simulink model "Control_Unit"  (R2023b)
settings: Solver=ode1  StartTime=0.0  StopTime=100  FixedStep=0.02  RelTol=1e-3  AbsTol=1e-3  EnableMultiTasking=on
model workspace: external: MATLAB File model_workspace.m (data not in the file)
values from neighbouring files (symbols this model uses):
  time_step = 0.02    [model_workspace.m]
libraries: slpidlib x3
settings Model: Creator=The MathWorks, Inc.  LastModifiedBy=danie
settings ConfigSet: Description=VeriStand Targets (Windows & NI Linux Real-Time 64-bit)
settings SolverCC: AutoScaleAbsTol=off  MaxConsecutiveMinStep=2  AlgebraicLoopSolver=TrustRegion  AutoInsertRateTranBlk=on  InsertRTBMode=Always  MaxZcPerStep=1
settings DataIOCC: SaveOutput=off  SaveTime=off  ReturnWorkspaceOutputs=off
settings OptimizationCC: DefaultParameterBehavior=Inlined  EnhancedBackFolding=on  PassReuseOutputArgsAs=Individual arguments  ZeroExternalMemoryAtStartup=off  ZeroInternalMemoryAtStartup=off  OptimizeBlockOrder=speed  DifferentSizesBufferReuse=on  OptimizationCustomize=off  EfficientTunableParamExpr=on
settings DebuggingCC: ParameterTunabilityLossMsg=error  UnconnectedInputMsg=warning  UnconnectedOutputMsg=warning  UnconnectedLineMsg=warning  SymbolicDimsDataTypeCodeGenerationDiagnostic=none
settings HardwareCC: ProdBitPerLong=64  ProdHWDeviceType=Intel->x86-64 (Linux 64)
settings ModelReferenceCC: EnableRefExpFcnMdlSchedulingChecks=on
settings SFSimCC: MATLABDynamicMemAlloc=off  CustomCodeUndefinedFunction=UseInterfaceOnly
settings RTWCC: Description=Embedded Coder  SystemTargetFile=ert.tlc  GenCodeOnly=on  PackageGeneratedCodeAndArtifacts=on  TemplateMakefile=ert_default_tmf  BuildConfiguration=Faster Runs  DLArmComputeVersion=19.05
settings CodeAppCC: ForceParamTrailComments=on  IgnoreCustomStorageClasses=off  OperatorAnnotations=on  SimulinkDataObjDesc=on  SFDataObjDesc=on  InsertBlockDesc=on
settings ERTTargetCC: TargetLangStandard=C99 (ISO)  GenerateSampleERTMain=on  InlinedParameterPlacement=NonHierarchical  ERTCustomFileTemplate=example_file_process.tlc
settings SimscapeCC: SimscapeLogType=all  SimscapeLogSimulationStatistics=on  SimscapeLogName=simlog_ssc_fuel_cell  SimscapeLogDataHistory=20000

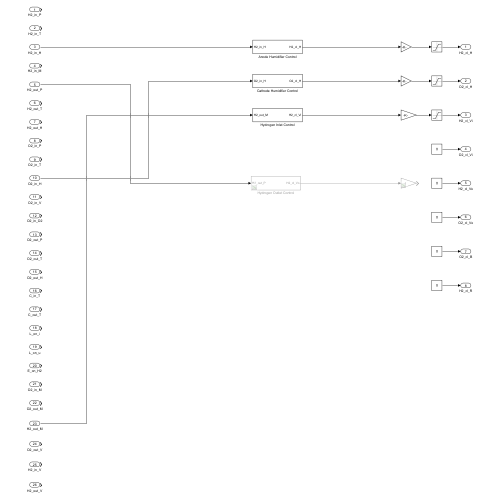
[thumbnail: Simulink's stored preview of the top-level diagram]
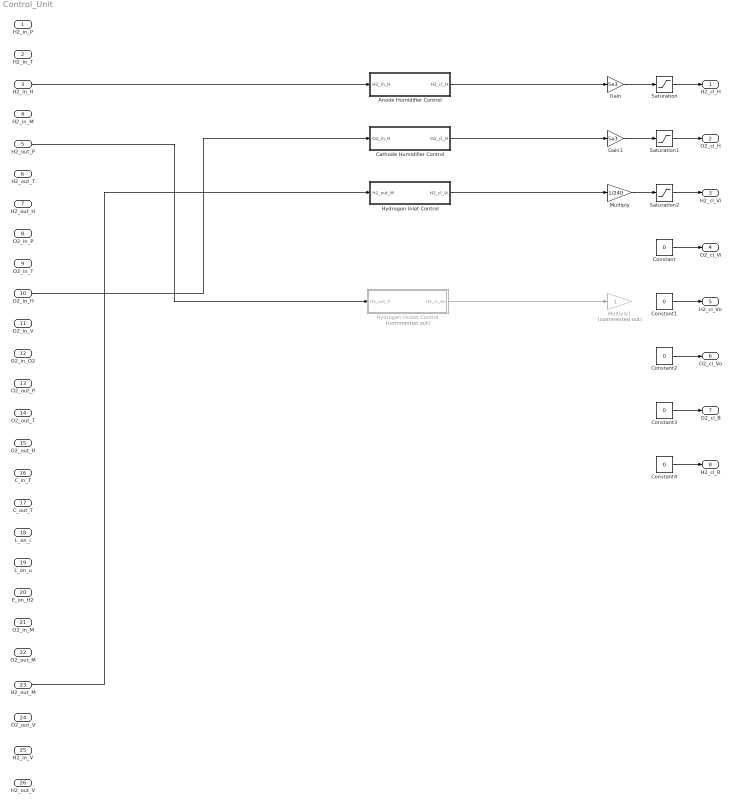
== system Control_Unit ==
  H2_in_P : Inport  OutDataTypeStr=double  PortDimensions=[1 1]  SampleTime=[time_step,0]
  H2_in_T : Inport  Port=2  OutDataTypeStr=double  PortDimensions=[1 1]  SampleTime=[time_step,0]
  H2_in_H : Inport  Port=3  OutDataTypeStr=double  PortDimensions=[1 1]  SampleTime=[time_step,0]
  H2_in_M : Inport  Port=4  OutDataTypeStr=double  PortDimensions=[1 1]  SampleTime=[time_step,0]
  H2_out_P : Inport  Port=5  OutDataTypeStr=double  PortDimensions=[1 1]  SampleTime=[time_step,0]
  H2_out_T : Inport  Port=6  OutDataTypeStr=double  PortDimensions=[1 1]  SampleTime=[time_step,0]
  H2_out_H : Inport  Port=7  OutDataTypeStr=double  PortDimensions=[1 1]  SampleTime=[time_step,0]
  O2_in_P : Inport  Port=8  OutDataTypeStr=double  PortDimensions=[1 1]  SampleTime=[time_step,0]
  O2_in_T : Inport  Port=9  OutDataTypeStr=double  PortDimensions=[1 1]  SampleTime=[time_step,0]
  O2_in_H : Inport  Port=10  OutDataTypeStr=double  PortDimensions=[1 1]  SampleTime=[time_step,0]
  O2_in_V : Inport  Port=11  OutDataTypeStr=double  PortDimensions=[1 1]  SampleTime=[time_step,0]
  O2_in_O2 : Inport  Port=12  OutDataTypeStr=double  PortDimensions=[1 1]  SampleTime=[time_step,0]
  O2_out_P : Inport  Port=13  OutDataTypeStr=double  PortDimensions=[1 1]  SampleTime=[time_step,0]
  O2_out_T : Inport  Port=14  OutDataTypeStr=double  PortDimensions=[1 1]  SampleTime=[time_step,0]
  O2_out_H : Inport  Port=15  OutDataTypeStr=double  PortDimensions=[1 1]  SampleTime=[time_step,0]
  C_in_T : Inport  Port=16  OutDataTypeStr=double  PortDimensions=1  SampleTime=[time_step,0]
  C_out_T : Inport  Port=17  OutDataTypeStr=double  PortDimensions=1  SampleTime=[time_step,0]
  L_on_i : Inport  Port=18  OutDataTypeStr=double  PortDimensions=1  SampleTime=[time_step,0]
  L_on_u : Inport  Port=19  OutDataTypeStr=double  PortDimensions=1  SampleTime=[time_step,0]
  E_on_H2 : Inport  Port=20  OutDataTypeStr=double  PortDimensions=1  SampleTime=[time_step,0]
  O2_in_M : Inport  Port=21  OutDataTypeStr=double  PortDimensions=[1 1]  SampleTime=[time_step,0]
  O2_out_M : Inport  Port=22  OutDataTypeStr=double  PortDimensions=[1 1]  SampleTime=[time_step,0]
  H2_out_M : Inport  Port=23  OutDataTypeStr=double  PortDimensions=[1 1]  SampleTime=[time_step,0]
  O2_out_V : Inport  Port=24  OutDataTypeStr=double  PortDimensions=[1 1]  SampleTime=[time_step,0]
  H2_in_V : Inport  Port=25  OutDataTypeStr=double  PortDimensions=[1 1]  SampleTime=[time_step,0]
  H2_out_V : Inport  Port=26  OutDataTypeStr=double  PortDimensions=[1 1]  SampleTime=[time_step,0]
  Anode Humidifier Control : Subsystem
  Cathode Humidifier Control : Subsystem
  Constant{,1..4} (5 alike) : Constant  Value=0
  Gain : Gain  Gain=5e3
  Gain1 : Gain  Gain=5e3
  Hydrogen Inlet Control : Subsystem
  Hydrogen Outlet Control : Subsystem  Commented=on
  Multiply : Gain  Gain=1/240
  Multiply1 : Gain  Commented=on
  Saturation : Saturate  UpperLimit=1  LowerLimit=0
  Saturation1 : Saturate  UpperLimit=1  LowerLimit=0
  Saturation2 : Saturate  UpperLimit=1  LowerLimit=0
  H2_cl_H : Outport  OutDataTypeStr=double  PortDimensions=[1 1]  SampleTime=[time_step,0]
  O2_cl_H : Outport  Port=2  OutDataTypeStr=double  PortDimensions=[1 1]  SampleTime=[time_step,0]
  H2_cl_Vi : Outport  Port=3  OutDataTypeStr=double  PortDimensions=1  SampleTime=[time_step,0]
  O2_cl_Vi : Outport  Port=4  OutDataTypeStr=double  PortDimensions=1  SampleTime=[time_step,0]
  H2_cl_Vo : Outport  Port=5  OutDataTypeStr=double  PortDimensions=1  SampleTime=[time_step,0]
  O2_cl_Vo : Outport  Port=6  OutDataTypeStr=double  PortDimensions=1  SampleTime=[time_step,0]
  O2_cl_B : Outport  Port=7  OutDataTypeStr=double  PortDimensions=1  SampleTime=[time_step,0]
  H2_cl_R : Outport  Port=8  OutDataTypeStr=double  PortDimensions=1  SampleTime=[time_step,0]
  wires:
  H2_in_H/1 -> Anode Humidifier Control/1(H2_in_H)
  O2_in_H/1 -> Cathode Humidifier Control/1(O2_in_H)
  Cathode Humidifier Control/1(O2_cl_H) -> Gain1/1
  Anode Humidifier Control/1(H2_cl_H) -> Gain/1
  Gain1/1 -> Saturation1/1
  Gain/1 -> Saturation/1
  Saturation1/1 -> O2_cl_H/1
  Saturation/1 -> H2_cl_H/1
  Multiply/1 -> Saturation2/1
  Saturation2/1 -> H2_cl_Vi/1
  Hydrogen Inlet Control/1(H2_cl_Vi) -> Multiply/1
  Constant/1 -> O2_cl_Vi/1
  H2_out_P/1 -> Hydrogen Outlet Control/1(H2_out_P)
  Constant2/1 -> O2_cl_Vo/1
  Constant3/1 -> O2_cl_B/1
  Constant4/1 -> H2_cl_R/1
  Hydrogen Outlet Control/1(H2_cl_Vo) -> Multiply1/1
  H2_out_M/1 -> Hydrogen Inlet Control/1(H2_out_M)
  Constant1/1 -> H2_cl_Vo/1

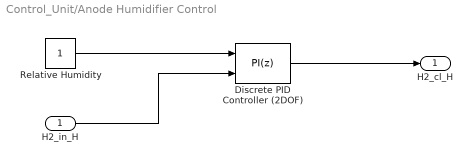
== system Control_Unit/Anode Humidifier Control ==
  H2_in_H : Inport
  Discrete PID Controller (2DOF) : slpidlib/PID Controller (2DOF)  Controller=PI  Form=Parallel  TimeDomain=Discrete-time  UseExternalTs=off  SampleTime=-1  IntegratorMethod=Forward Euler  FilterMethod=Forward Euler  ControllerParametersSource=internal  P=0.0001  I=0.001  UseKiTs=off  D=0  N=100  UseFilter=on  b=1  c=1  TunerSelectOption=Transfer Function Based (PID Tuner App)  InitialConditionSource=internal  InitialConditionForIntegrator=0  InitialConditionForFilter=0  DifferentiatorICPrevScaledInput=0  ExternalReset=none  TrackingMode=off  Kt=1  LimitOutput=on  SatLimitsSource=internal  UpperSaturationLimit=.2e-3  LowerSaturationLimit=0  LinearizeAsGain=off  AntiWindupMode=clamping  Kb=1  LimitIntegrator=off  UpperIntegratorSaturationLimit=inf  LowerIntegratorSaturationLimit=-inf  POutMin=[]  POutMax=[]  IOutMin=[]  IOutMax=[]  DOutMin=[]  DOutMax=[]  NOutMin=[]  NOutMax=[]  bOutMin=[]  bOutMax=[]  cOutMin=[]  cOutMax=[]  SumOutMin=[]  SumOutMax=[]  SaturationOutMin=[]  SaturationOutMax=[]  PParamMin=[]  PParamMax=[]  IParamMin=[]  IParamMax=[]  DParamMin=[]  DParamMax=[]  NParamMin=[]  NParamMax=[]  bParamMin=[]  bParamMax=[]  cParamMin=[]  cParamMax=[]  KbParamMin=[]  KbParamMax=[]  KtParamMin=[]  KtParamMax=[]  KbOutMin=[]  KbOutMax=[]  KtOutMin=[]  KtOutMax=[]  IntegratorOutMin=[]  IntegratorOutMax=[]  FilterOutMin=[]  FilterOutMax=[]  SumI1OutMin=[]  SumI1OutMax=[]  SumI2OutMin=[]  SumI2OutMax=[]  SumI3OutMin=[]  SumI3OutMax=[]  SumI4OutMin=[]  SumI4OutMax=[]  SumDOutMin=[]  SumDOutMax=[]  Sum1OutMin=[]  Sum1OutMax=[]  Sum2OutMin=[]  Sum2OutMax=[]  Sum3OutMin=[]  Sum3OutMax=[]  DifferentiatorOutMin=[]  DifferentiatorOutMax=[]  FilterDiffOutCoefMin=[]  FilterDiffOutCoefMax=[]  ReciprocalOutMin=[]  ReciprocalOutMax=[]  SumDenOutMin=[]  SumDenOutMax=[]  SumNumOutMin=[]  SumNumOutMax=[]  DivideOutMin=[]  DivideOutMax=[]  UdiffTsProdOutMin=[]  UdiffTsProdOutMax=[]  NTsProdOutMin=[]  NTsProdOutMax=[]  UintegralTsProdOutMin=[]  UintegralTsProdOutMax=[]  UngainTsProdOutMin=[]  UngainTsProdOutMax=[]  ClampingZeroOutDataTypeStr=Inherit: Inherit via back propagation  ClampingZeroOutMin=[]  ClampingZeroOutMax=[]  FilterDenConstantOutDataTypeStr=Inherit: Inherit via back propagation  FilterDenConstantOutMin=[]  FilterDenConstantOutMax=[]  PCopyOutDataTypeStr=Inherit: Inherit via back propagation  PCopyOutMin=[]  PCopyOutMax=[]  NCopyOutDataTypeStr=Inherit: Inherit via back propagation  NCopyOutMin=[]  NCopyOutMax=[]  IntegratorContinuousStateAttributes=''  IntegratorStateMustResolveToSignalObject=off  IntegratorRTWStateStorageClass=Auto  FilterContinuousStateAttributes=''  FilterStateMustResolveToSignalObject=off  FilterRTWStateStorageClass=Auto  ParallelPVariant=InternalParameters  IdealPVariant=Disabled  IVariant=InternalParameters  DVariant=Disabled  bVariant=InternalParameters  cVariant=Disabled  IntegratorVariant=Discrete  SatVariant=Enabled  AWVariant=DiscClampingParallel  PCopyVariant=Disabled  TRVariant=Disabled  FdbkBlocksVariant=Forward  IdealPFdbkVariant=Disabled  SatFdbkVariant=Disabled  DerivativeFilterVariant=Disabled  NVariant=Disabled  NCopyVariant=Disabled_SignalSpec  FilterICVariant=Disabled  IntegratorICVariant=InternalICs  ExternalResetVariant=Disabled  TRSumVariant=Passthrough  SumFdbkVariant=Disabled  SumVariant=Sum_PI  TsampFilterVariant=InternalTs  TsampNgainVariant=Passthrough  TsampIntegralVariant=Disabled_SignalSpec  ExternalSaturationOutDataTypeStr=Inherit: Same as second input
  Relative Humidity : Constant
  H2_cl_H : Outport
  wires:
  Relative Humidity/1 -> Discrete PID Controller (2DOF)/1
  H2_in_H/1 -> Discrete PID Controller (2DOF)/2
  Discrete PID Controller (2DOF)/1 -> H2_cl_H/1

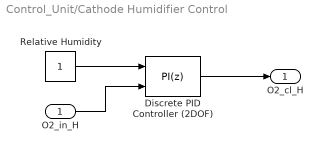
== system Control_Unit/Cathode Humidifier Control ==
  O2_in_H : Inport
  Discrete PID Controller (2DOF) : slpidlib/PID Controller (2DOF)  Controller=PI  Form=Parallel  TimeDomain=Discrete-time  UseExternalTs=off  SampleTime=-1  IntegratorMethod=Forward Euler  FilterMethod=Forward Euler  ControllerParametersSource=internal  P=0.0001  I=0.001  UseKiTs=off  D=0  N=100  UseFilter=on  b=1  c=1  TunerSelectOption=Transfer Function Based (PID Tuner App)  InitialConditionSource=internal  InitialConditionForIntegrator=0  InitialConditionForFilter=0  DifferentiatorICPrevScaledInput=0  ExternalReset=none  TrackingMode=off  Kt=1  LimitOutput=on  SatLimitsSource=internal  UpperSaturationLimit=.2e-3  LowerSaturationLimit=0  LinearizeAsGain=off  AntiWindupMode=clamping  Kb=1  LimitIntegrator=off  UpperIntegratorSaturationLimit=inf  LowerIntegratorSaturationLimit=-inf  POutMin=[]  POutMax=[]  IOutMin=[]  IOutMax=[]  DOutMin=[]  DOutMax=[]  NOutMin=[]  NOutMax=[]  bOutMin=[]  bOutMax=[]  cOutMin=[]  cOutMax=[]  SumOutMin=[]  SumOutMax=[]  SaturationOutMin=[]  SaturationOutMax=[]  PParamMin=[]  PParamMax=[]  IParamMin=[]  IParamMax=[]  DParamMin=[]  DParamMax=[]  NParamMin=[]  NParamMax=[]  bParamMin=[]  bParamMax=[]  cParamMin=[]  cParamMax=[]  KbParamMin=[]  KbParamMax=[]  KtParamMin=[]  KtParamMax=[]  KbOutMin=[]  KbOutMax=[]  KtOutMin=[]  KtOutMax=[]  IntegratorOutMin=[]  IntegratorOutMax=[]  FilterOutMin=[]  FilterOutMax=[]  SumI1OutMin=[]  SumI1OutMax=[]  SumI2OutMin=[]  SumI2OutMax=[]  SumI3OutMin=[]  SumI3OutMax=[]  SumI4OutMin=[]  SumI4OutMax=[]  SumDOutMin=[]  SumDOutMax=[]  Sum1OutMin=[]  Sum1OutMax=[]  Sum2OutMin=[]  Sum2OutMax=[]  Sum3OutMin=[]  Sum3OutMax=[]  DifferentiatorOutMin=[]  DifferentiatorOutMax=[]  FilterDiffOutCoefMin=[]  FilterDiffOutCoefMax=[]  ReciprocalOutMin=[]  ReciprocalOutMax=[]  SumDenOutMin=[]  SumDenOutMax=[]  SumNumOutMin=[]  SumNumOutMax=[]  DivideOutMin=[]  DivideOutMax=[]  UdiffTsProdOutMin=[]  UdiffTsProdOutMax=[]  NTsProdOutMin=[]  NTsProdOutMax=[]  UintegralTsProdOutMin=[]  UintegralTsProdOutMax=[]  UngainTsProdOutMin=[]  UngainTsProdOutMax=[]  ClampingZeroOutDataTypeStr=Inherit: Inherit via back propagation  ClampingZeroOutMin=[]  ClampingZeroOutMax=[]  FilterDenConstantOutDataTypeStr=Inherit: Inherit via back propagation  FilterDenConstantOutMin=[]  FilterDenConstantOutMax=[]  PCopyOutDataTypeStr=Inherit: Inherit via back propagation  PCopyOutMin=[]  PCopyOutMax=[]  NCopyOutDataTypeStr=Inherit: Inherit via back propagation  NCopyOutMin=[]  NCopyOutMax=[]  IntegratorContinuousStateAttributes=''  IntegratorStateMustResolveToSignalObject=off  IntegratorRTWStateStorageClass=Auto  FilterContinuousStateAttributes=''  FilterStateMustResolveToSignalObject=off  FilterRTWStateStorageClass=Auto  ParallelPVariant=InternalParameters  IdealPVariant=Disabled  IVariant=InternalParameters  DVariant=Disabled  bVariant=InternalParameters  cVariant=Disabled  IntegratorVariant=Discrete  SatVariant=Enabled  AWVariant=DiscClampingParallel  PCopyVariant=Disabled  TRVariant=Disabled  FdbkBlocksVariant=Forward  IdealPFdbkVariant=Disabled  SatFdbkVariant=Disabled  DerivativeFilterVariant=Disabled  NVariant=Disabled  NCopyVariant=Disabled_SignalSpec  FilterICVariant=Disabled  IntegratorICVariant=InternalICs  ExternalResetVariant=Disabled  TRSumVariant=Passthrough  SumFdbkVariant=Disabled  SumVariant=Sum_PI  TsampFilterVariant=InternalTs  TsampNgainVariant=Passthrough  TsampIntegralVariant=Disabled_SignalSpec  ExternalSaturationOutDataTypeStr=Inherit: Same as second input
  Relative Humidity : Constant
  O2_cl_H : Outport
  wires:
  Discrete PID Controller (2DOF)/1 -> O2_cl_H/1
  Relative Humidity/1 -> Discrete PID Controller (2DOF)/1
  O2_in_H/1 -> Discrete PID Controller (2DOF)/2

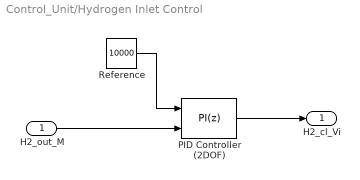
== system Control_Unit/Hydrogen Inlet Control ==
  H2_out_M : Inport
  PID Controller (2DOF) : slpidlib/PID Controller (2DOF)  Controller=PI  Form=Parallel  TimeDomain=Discrete-time  UseExternalTs=off  SampleTime=-1  IntegratorMethod=Forward Euler  FilterMethod=Forward Euler  ControllerParametersSource=internal  P=0  I=0.01  UseKiTs=off  D=0  N=100  UseFilter=on  b=1  c=1  TunerSelectOption=Transfer Function Based (PID Tuner App)  InitialConditionSource=internal  InitialConditionForIntegrator=0  InitialConditionForFilter=0  DifferentiatorICPrevScaledInput=0  ExternalReset=none  TrackingMode=off  Kt=1  LimitOutput=on  SatLimitsSource=internal  UpperSaturationLimit=240  LowerSaturationLimit=0  LinearizeAsGain=on  AntiWindupMode=back-calculation  Kb=1  LimitIntegrator=off  UpperIntegratorSaturationLimit=inf  LowerIntegratorSaturationLimit=-inf  POutMin=[]  POutMax=[]  IOutMin=[]  IOutMax=[]  DOutMin=[]  DOutMax=[]  NOutMin=[]  NOutMax=[]  bOutMin=[]  bOutMax=[]  cOutMin=[]  cOutMax=[]  SumOutMin=[]  SumOutMax=[]  SaturationOutMin=[]  SaturationOutMax=[]  PParamMin=[]  PParamMax=[]  IParamMin=[]  IParamMax=[]  DParamMin=[]  DParamMax=[]  NParamMin=[]  NParamMax=[]  bParamMin=[]  bParamMax=[]  cParamMin=[]  cParamMax=[]  KbParamMin=[]  KbParamMax=[]  KtParamMin=[]  KtParamMax=[]  KbOutMin=[]  KbOutMax=[]  KtOutMin=[]  KtOutMax=[]  IntegratorOutMin=[]  IntegratorOutMax=[]  FilterOutMin=[]  FilterOutMax=[]  SumI1OutMin=[]  SumI1OutMax=[]  SumI2OutMin=[]  SumI2OutMax=[]  SumI3OutMin=[]  SumI3OutMax=[]  SumI4OutMin=[]  SumI4OutMax=[]  SumDOutMin=[]  SumDOutMax=[]  Sum1OutMin=[]  Sum1OutMax=[]  Sum2OutMin=[]  Sum2OutMax=[]  Sum3OutMin=[]  Sum3OutMax=[]  DifferentiatorOutMin=[]  DifferentiatorOutMax=[]  FilterDiffOutCoefMin=[]  FilterDiffOutCoefMax=[]  ReciprocalOutMin=[]  ReciprocalOutMax=[]  SumDenOutMin=[]  SumDenOutMax=[]  SumNumOutMin=[]  SumNumOutMax=[]  DivideOutMin=[]  DivideOutMax=[]  UdiffTsProdOutMin=[]  UdiffTsProdOutMax=[]  NTsProdOutMin=[]  NTsProdOutMax=[]  UintegralTsProdOutMin=[]  UintegralTsProdOutMax=[]  UngainTsProdOutMin=[]  UngainTsProdOutMax=[]  ClampingZeroOutDataTypeStr=Inherit: Inherit via back propagation  ClampingZeroOutMin=[]  ClampingZeroOutMax=[]  FilterDenConstantOutDataTypeStr=Inherit: Inherit via back propagation  FilterDenConstantOutMin=[]  FilterDenConstantOutMax=[]  PCopyOutDataTypeStr=Inherit: Inherit via back propagation  PCopyOutMin=[]  PCopyOutMax=[]  NCopyOutDataTypeStr=Inherit: Inherit via back propagation  NCopyOutMin=[]  NCopyOutMax=[]  IntegratorContinuousStateAttributes=''  IntegratorStateMustResolveToSignalObject=off  IntegratorRTWStateStorageClass=Auto  FilterContinuousStateAttributes=''  FilterStateMustResolveToSignalObject=off  FilterRTWStateStorageClass=Auto  ParallelPVariant=InternalParameters  IdealPVariant=Disabled  IVariant=InternalParameters  DVariant=Disabled  bVariant=InternalParameters  cVariant=Disabled  IntegratorVariant=Discrete  SatVariant=Enabled  AWVariant=BackCalculation  PCopyVariant=Disabled  TRVariant=Disabled  FdbkBlocksVariant=Forward  IdealPFdbkVariant=Disabled  SatFdbkVariant=Disabled  DerivativeFilterVariant=Disabled  NVariant=Disabled  NCopyVariant=Disabled_SignalSpec  FilterICVariant=Disabled  IntegratorICVariant=InternalICs  ExternalResetVariant=Disabled  TRSumVariant=Passthrough  SumFdbkVariant=Disabled  SumVariant=Sum_PI  TsampFilterVariant=InternalTs  TsampNgainVariant=Passthrough  TsampIntegralVariant=Disabled_SignalSpec  ExternalSaturationOutDataTypeStr=Inherit: Same as second input
  Reference : Constant  Value=10000
  H2_cl_Vi : Outport
  wires:
  PID Controller (2DOF)/1 -> H2_cl_Vi/1
  Reference/1 -> PID Controller (2DOF)/1
  H2_out_M/1 -> PID Controller (2DOF)/2

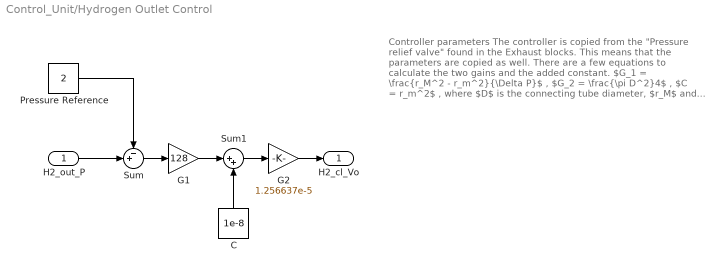
== system Control_Unit/Hydrogen Outlet Control ==
  note: Controller parameters
      |
      | The controller is copied from the "Pressure relief valve" found in the Exhaust blocks.
      |
      | This means that the parameters are copied as well. There are a few equations to calculate the two gains and the added constant.
      |
      | $G_1 = \frac{r_M^2 - r_m^2}{\Delta P}$ , $G_2 = \frac{\pi D^2}4$ , $C = r_m^2$ ,
      |
      | where $D$ is the connecting tube diameter, $r_M$ and $r_m$ are the maximal and minimal diameter ratios, while $\Delta P$ is the pressure regulation range.
  H2_out_P : Inport
  C : Constant  Value=1e-8
  G1 : Gain  Gain=128
  G2 : Gain  Gain=1.256637e-5
  Pressure Reference : Constant  Value=2
  Sum : Sum  Inputs=-+|
  Sum1 : Sum  Inputs=|++
  H2_cl_Vo : Outport
  wires:
  Pressure Reference/1 -> Sum/1
  H2_out_P/1 -> Sum/2
  Sum/1 -> G1/1
  G1/1 -> Sum1/1
  C/1 -> Sum1/2
  Sum1/1 -> G2/1
  G2/1 -> H2_cl_Vo/1
